simulink model "wheelPWM"  (R2018a)
settings: Solver=VariableStepAuto  StartTime=0.0  StopTime=10.0  RelTol=1e-3
settings Model: Creator=wangkingsheng  LastModifiedBy=wangkingsheng

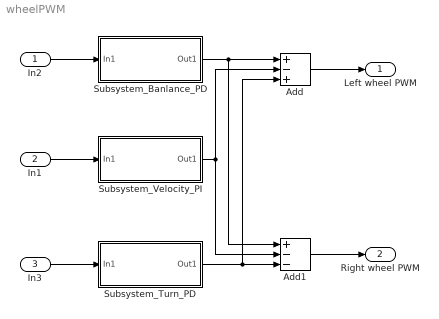
== system wheelPWM ==
  In2 : Inport
  In1 : Inport  Port=2
  In3 : Inport  Port=3
  Add : Sum  Inputs=+-+
  Add1 : Sum  Inputs=+--
  Subsystem_Banlance_PD : Subsystem
  Subsystem_Turn_PD : Subsystem
  Subsystem_Velocity_PI : Subsystem
  Left wheel PWM : Outport
  Right wheel PWM : Outport  Port=2
  wires:
  In2/1 -> Subsystem_Banlance_PD/1(In1)
  In1/1 -> Subsystem_Velocity_PI/1(In1)
  In3/1 -> Subsystem_Turn_PD/1(In1)
  Add/1 -> Left wheel PWM/1
  Add1/1 -> Right wheel PWM/1
  Subsystem_Turn_PD/1(Out1) -> Add/3, Add1/3
  Subsystem_Banlance_PD/1(Out1) -> Add1/1, Add/1
  Subsystem_Velocity_PI/1(Out1) -> Add1/2, Add/2

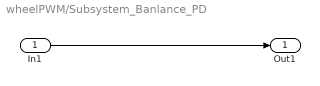
== system wheelPWM/Subsystem_Banlance_PD ==
  In1 : Inport
  Out1 : Outport
  wires:
  In1/1 -> Out1/1

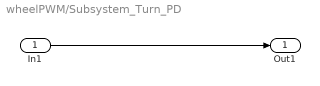
== system wheelPWM/Subsystem_Turn_PD ==
  In1 : Inport
  Out1 : Outport
  wires:
  In1/1 -> Out1/1

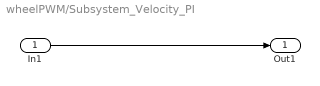
== system wheelPWM/Subsystem_Velocity_PI ==
  In1 : Inport
  Out1 : Outport
  wires:
  In1/1 -> Out1/1
